simulink model "simulink_controll_attitude_5kg"  (R2015a)
settings: Solver=ode45  StartTime=0.0  StopTime=40  RelTol=1e-3
libraries: fuzblock x4
settings Model: Creator=Marcos  LastModifiedBy=Marcos

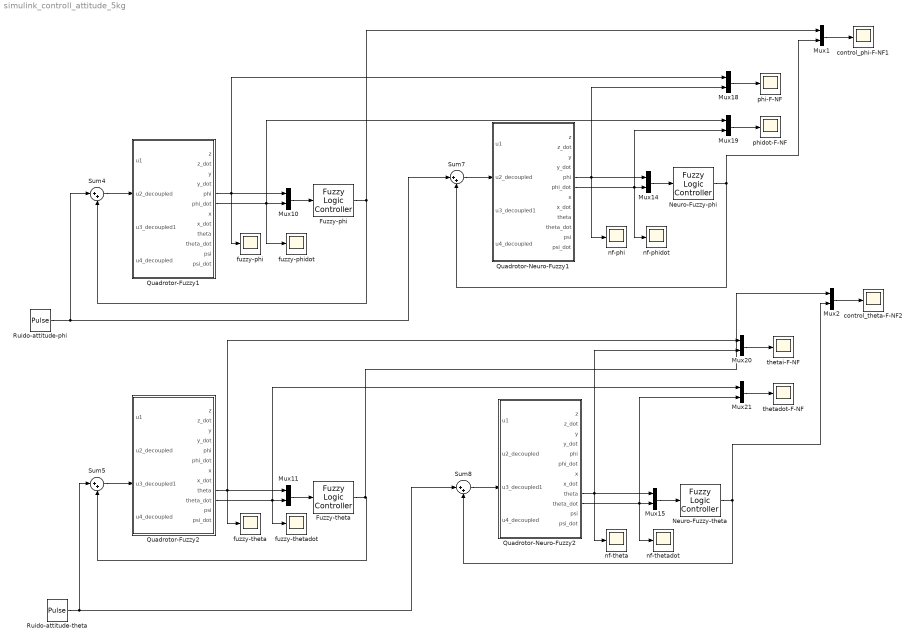
== system simulink_controll_attitude_5kg ==
  Fuzzy-phi : fuzblock/Fuzzy Logic  Controller  fis='fis_attitude.fis'
  Fuzzy-theta : fuzblock/Fuzzy Logic  Controller  fis='fis_attitude.fis'
  Mux{1..2,10..11,14..15,18..21} (10 alike) : Mux  Inputs=2
  Neuro-Fuzzy-phi : fuzblock/Fuzzy Logic  Controller  fis='anfis_attitude.fis'
  Neuro-Fuzzy-theta : fuzblock/Fuzzy Logic  Controller  fis='anfis_attitude.fis'
  Quadrotor-Fuzzy1 : Subsystem
  Quadrotor-Fuzzy2 : Subsystem
  Quadrotor-Neuro-Fuzzy1 : Subsystem
  Quadrotor-Neuro-Fuzzy2 : Subsystem
  Ruido-attitude-phi : DiscretePulseGenerator  PulseType=Time based  Amplitude=20  Period=40  PulseWidth=0.05
  Ruido-attitude-theta : DiscretePulseGenerator  PulseType=Time based  Amplitude=20  Period=40  PulseWidth=0.05
  Sum{4..5,7..8} (4 alike) : Sum  Inputs=|++
  control_phi-F-NF1 : Scope
      settings: SaveName=control_phi5
  control_theta-F-NF2 : Scope
      settings: SaveName=control_theta5
  fuzzy-phi : Scope
      settings: SaveName=ScopeData19
  fuzzy-phidot : Scope
      settings: SaveName=ScopeData20
  fuzzy-theta : Scope
      settings: SaveName=ScopeData21
  fuzzy-thetadot : Scope
      settings: SaveName=ScopeData22
  nf-phi : Scope
      settings: SaveName=ScopeData25
  nf-phidot : Scope
      settings: SaveName=ScopeData26
  nf-theta : Scope
      settings: SaveName=ScopeData27
  nf-thetadot : Scope
      settings: SaveName=ScopeData28
  phi-F-NF : Scope
      settings: SaveName=phi5
  phidot-F-NF : Scope
      settings: SaveName=phidot5
  thetadot-F-NF : Scope
      settings: SaveName=thetadot5
  thetai-F-NF : Scope
      settings: SaveName=theta5
  wires:
  Mux10/1 -> Fuzzy-phi/1
  Quadrotor-Fuzzy1/5(phi) -> Mux18/1, fuzzy-phi/1, Mux10/1
  Sum4/1 -> Quadrotor-Fuzzy1/2(u2_decoupled)
  Fuzzy-phi/1 -> Sum4/2, Mux1/1
  Quadrotor-Fuzzy1/6(phi_dot) -> Mux19/1, fuzzy-phidot/1, Mux10/2
  Quadrotor-Fuzzy2/9(theta) -> Mux20/1, fuzzy-theta/1, Mux11/1
  Sum5/1 -> Quadrotor-Fuzzy2/3(u3_decoupled1)
  Fuzzy-theta/1 -> Mux2/1, Sum5/2
  Quadrotor-Fuzzy2/10(theta_dot) -> fuzzy-thetadot/1, Mux21/1, Mux11/2
  Mux11/1 -> Fuzzy-theta/1
  Mux14/1 -> Neuro-Fuzzy-phi/1
  Ruido-attitude-phi/1 -> Sum7/1, Sum4/1
  Quadrotor-Neuro-Fuzzy1/5(phi) -> Mux18/2, nf-phi/1, Mux14/1
  Sum7/1 -> Quadrotor-Neuro-Fuzzy1/2(u2_decoupled)
  Neuro-Fuzzy-phi/1 -> Mux1/2, Sum7/2
  Quadrotor-Neuro-Fuzzy1/6(phi_dot) -> Mux19/2, nf-phidot/1, Mux14/2
  Ruido-attitude-theta/1 -> Sum8/1, Sum5/1
  Quadrotor-Neuro-Fuzzy2/9(theta) -> Mux20/2, nf-theta/1, Mux15/1
  Sum8/1 -> Quadrotor-Neuro-Fuzzy2/3(u3_decoupled1)
  Neuro-Fuzzy-theta/1 -> Mux2/2, Sum8/2
  Quadrotor-Neuro-Fuzzy2/10(theta_dot) -> Mux21/2, nf-thetadot/1, Mux15/2
  Mux15/1 -> Neuro-Fuzzy-theta/1
  Mux20/1 -> thetai-F-NF/1
  Mux21/1 -> thetadot-F-NF/1
  Mux18/1 -> phi-F-NF/1
  Mux19/1 -> phidot-F-NF/1
  Mux1/1 -> control_phi-F-NF1/1
  Mux2/1 -> control_theta-F-NF2/1

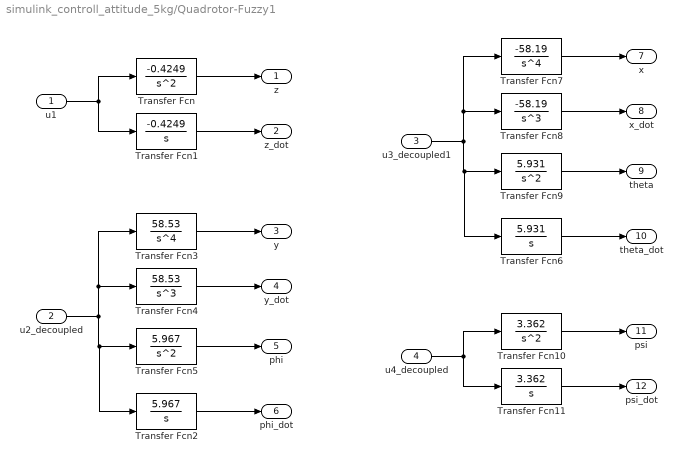
== system simulink_controll_attitude_5kg/Quadrotor-Fuzzy1 ==
  u1 : Inport
  u2_decoupled : Inport  Port=2
  u3_decoupled1 : Inport  Port=3
  u4_decoupled : Inport  Port=4
  Transfer Fcn : TransferFcn  Numerator=[-0.4249]  Denominator=[1 0 0]
  Transfer Fcn1 : TransferFcn  Numerator=[-0.4249]  Denominator=[1 0]
  Transfer Fcn10 : TransferFcn  Numerator=[3.362]  Denominator=[1 0 0]
  Transfer Fcn11 : TransferFcn  Numerator=[3.362]  Denominator=[1 0]
  Transfer Fcn2 : TransferFcn  Numerator=[5.967]  Denominator=[1 0]
  Transfer Fcn3 : TransferFcn  Numerator=[58.53]  Denominator=[1 0 0 0 0]
  Transfer Fcn4 : TransferFcn  Numerator=[58.53]  Denominator=[1 0 0 0]
  Transfer Fcn5 : TransferFcn  Numerator=[5.967]  Denominator=[1 0 0]
  Transfer Fcn6 : TransferFcn  Numerator=[5.931]  Denominator=[1 0]
  Transfer Fcn7 : TransferFcn  Numerator=[-58.19]  Denominator=[1 0 0 0 0]
  Transfer Fcn8 : TransferFcn  Numerator=[-58.19]  Denominator=[1 0 0 0]
  Transfer Fcn9 : TransferFcn  Numerator=[5.931]  Denominator=[1 0 0]
  z : Outport
  z_dot : Outport  Port=2
  y : Outport  Port=3
  y_dot : Outport  Port=4
  phi : Outport  Port=5
  phi_dot : Outport  Port=6
  x : Outport  Port=7
  x_dot : Outport  Port=8
  theta : Outport  Port=9
  theta_dot : Outport  Port=10
  psi : Outport  Port=11
  psi_dot : Outport  Port=12
  wires:
  Transfer Fcn/1 -> z/1
  u1/1 -> Transfer Fcn/1, Transfer Fcn1/1
  Transfer Fcn1/1 -> z_dot/1
  Transfer Fcn3/1 -> y/1
  u2_decoupled/1 -> Transfer Fcn3/1, Transfer Fcn4/1, Transfer Fcn2/1, Transfer Fcn5/1
  Transfer Fcn4/1 -> y_dot/1
  Transfer Fcn5/1 -> phi/1
  Transfer Fcn2/1 -> phi_dot/1
  Transfer Fcn7/1 -> x/1
  u3_decoupled1/1 -> Transfer Fcn7/1, Transfer Fcn8/1, Transfer Fcn6/1, Transfer Fcn9/1
  Transfer Fcn8/1 -> x_dot/1
  Transfer Fcn9/1 -> theta/1
  Transfer Fcn6/1 -> theta_dot/1
  Transfer Fcn10/1 -> psi/1
  u4_decoupled/1 -> Transfer Fcn10/1, Transfer Fcn11/1
  Transfer Fcn11/1 -> psi_dot/1

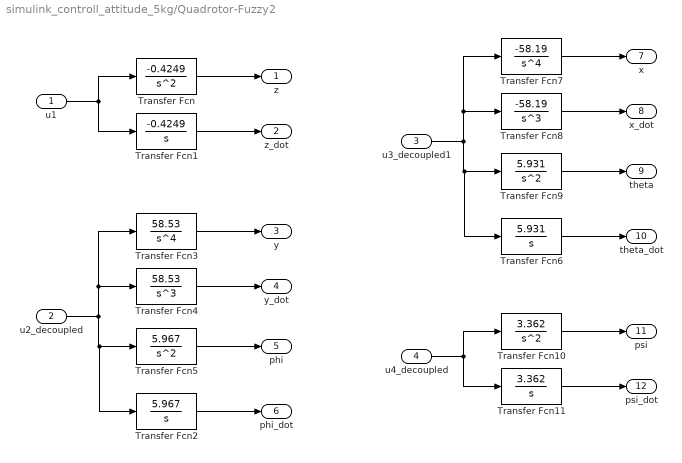
== system simulink_controll_attitude_5kg/Quadrotor-Fuzzy2 ==
  u1 : Inport
  u2_decoupled : Inport  Port=2
  u3_decoupled1 : Inport  Port=3
  u4_decoupled : Inport  Port=4
  Transfer Fcn : TransferFcn  Numerator=[-0.4249]  Denominator=[1 0 0]
  Transfer Fcn1 : TransferFcn  Numerator=[-0.4249]  Denominator=[1 0]
  Transfer Fcn10 : TransferFcn  Numerator=[3.362]  Denominator=[1 0 0]
  Transfer Fcn11 : TransferFcn  Numerator=[3.362]  Denominator=[1 0]
  Transfer Fcn2 : TransferFcn  Numerator=[5.967]  Denominator=[1 0]
  Transfer Fcn3 : TransferFcn  Numerator=[58.53]  Denominator=[1 0 0 0 0]
  Transfer Fcn4 : TransferFcn  Numerator=[58.53]  Denominator=[1 0 0 0]
  Transfer Fcn5 : TransferFcn  Numerator=[5.967]  Denominator=[1 0 0]
  Transfer Fcn6 : TransferFcn  Numerator=[5.931]  Denominator=[1 0]
  Transfer Fcn7 : TransferFcn  Numerator=[-58.19]  Denominator=[1 0 0 0 0]
  Transfer Fcn8 : TransferFcn  Numerator=[-58.19]  Denominator=[1 0 0 0]
  Transfer Fcn9 : TransferFcn  Numerator=[5.931]  Denominator=[1 0 0]
  z : Outport
  z_dot : Outport  Port=2
  y : Outport  Port=3
  y_dot : Outport  Port=4
  phi : Outport  Port=5
  phi_dot : Outport  Port=6
  x : Outport  Port=7
  x_dot : Outport  Port=8
  theta : Outport  Port=9
  theta_dot : Outport  Port=10
  psi : Outport  Port=11
  psi_dot : Outport  Port=12
  wires:
  Transfer Fcn/1 -> z/1
  u1/1 -> Transfer Fcn/1, Transfer Fcn1/1
  Transfer Fcn1/1 -> z_dot/1
  Transfer Fcn3/1 -> y/1
  u2_decoupled/1 -> Transfer Fcn3/1, Transfer Fcn4/1, Transfer Fcn2/1, Transfer Fcn5/1
  Transfer Fcn4/1 -> y_dot/1
  Transfer Fcn5/1 -> phi/1
  Transfer Fcn2/1 -> phi_dot/1
  Transfer Fcn7/1 -> x/1
  u3_decoupled1/1 -> Transfer Fcn7/1, Transfer Fcn8/1, Transfer Fcn6/1, Transfer Fcn9/1
  Transfer Fcn8/1 -> x_dot/1
  Transfer Fcn9/1 -> theta/1
  Transfer Fcn6/1 -> theta_dot/1
  Transfer Fcn10/1 -> psi/1
  u4_decoupled/1 -> Transfer Fcn10/1, Transfer Fcn11/1
  Transfer Fcn11/1 -> psi_dot/1

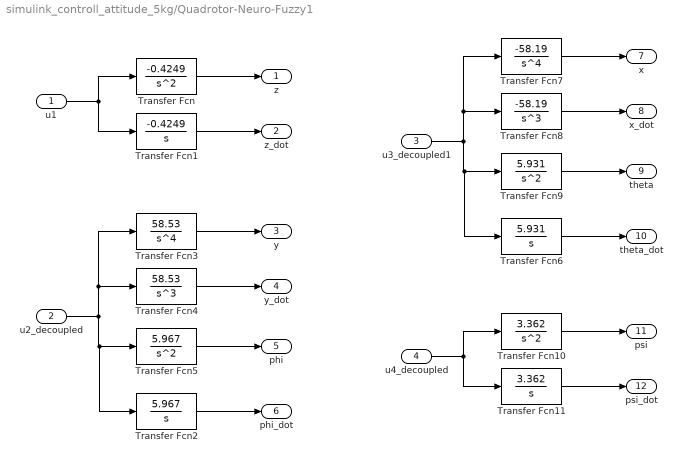
== system simulink_controll_attitude_5kg/Quadrotor-Neuro-Fuzzy1 ==
  u1 : Inport
  u2_decoupled : Inport  Port=2
  u3_decoupled1 : Inport  Port=3
  u4_decoupled : Inport  Port=4
  Transfer Fcn : TransferFcn  Numerator=[-0.4249]  Denominator=[1 0 0]
  Transfer Fcn1 : TransferFcn  Numerator=[-0.4249]  Denominator=[1 0]
  Transfer Fcn10 : TransferFcn  Numerator=[3.362]  Denominator=[1 0 0]
  Transfer Fcn11 : TransferFcn  Numerator=[3.362]  Denominator=[1 0]
  Transfer Fcn2 : TransferFcn  Numerator=[5.967]  Denominator=[1 0]
  Transfer Fcn3 : TransferFcn  Numerator=[58.53]  Denominator=[1 0 0 0 0]
  Transfer Fcn4 : TransferFcn  Numerator=[58.53]  Denominator=[1 0 0 0]
  Transfer Fcn5 : TransferFcn  Numerator=[5.967]  Denominator=[1 0 0]
  Transfer Fcn6 : TransferFcn  Numerator=[5.931]  Denominator=[1 0]
  Transfer Fcn7 : TransferFcn  Numerator=[-58.19]  Denominator=[1 0 0 0 0]
  Transfer Fcn8 : TransferFcn  Numerator=[-58.19]  Denominator=[1 0 0 0]
  Transfer Fcn9 : TransferFcn  Numerator=[5.931]  Denominator=[1 0 0]
  z : Outport
  z_dot : Outport  Port=2
  y : Outport  Port=3
  y_dot : Outport  Port=4
  phi : Outport  Port=5
  phi_dot : Outport  Port=6
  x : Outport  Port=7
  x_dot : Outport  Port=8
  theta : Outport  Port=9
  theta_dot : Outport  Port=10
  psi : Outport  Port=11
  psi_dot : Outport  Port=12
  wires:
  Transfer Fcn/1 -> z/1
  u1/1 -> Transfer Fcn/1, Transfer Fcn1/1
  Transfer Fcn1/1 -> z_dot/1
  Transfer Fcn3/1 -> y/1
  u2_decoupled/1 -> Transfer Fcn3/1, Transfer Fcn4/1, Transfer Fcn2/1, Transfer Fcn5/1
  Transfer Fcn4/1 -> y_dot/1
  Transfer Fcn5/1 -> phi/1
  Transfer Fcn2/1 -> phi_dot/1
  Transfer Fcn7/1 -> x/1
  u3_decoupled1/1 -> Transfer Fcn7/1, Transfer Fcn8/1, Transfer Fcn6/1, Transfer Fcn9/1
  Transfer Fcn8/1 -> x_dot/1
  Transfer Fcn9/1 -> theta/1
  Transfer Fcn6/1 -> theta_dot/1
  Transfer Fcn10/1 -> psi/1
  u4_decoupled/1 -> Transfer Fcn10/1, Transfer Fcn11/1
  Transfer Fcn11/1 -> psi_dot/1

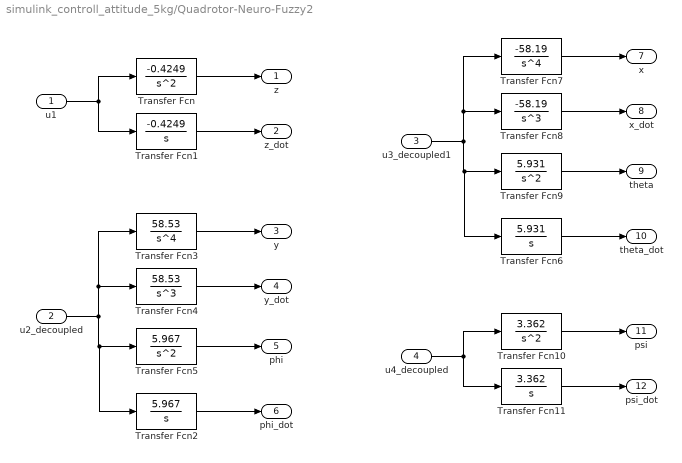
== system simulink_controll_attitude_5kg/Quadrotor-Neuro-Fuzzy2 ==
  u1 : Inport
  u2_decoupled : Inport  Port=2
  u3_decoupled1 : Inport  Port=3
  u4_decoupled : Inport  Port=4
  Transfer Fcn : TransferFcn  Numerator=[-0.4249]  Denominator=[1 0 0]
  Transfer Fcn1 : TransferFcn  Numerator=[-0.4249]  Denominator=[1 0]
  Transfer Fcn10 : TransferFcn  Numerator=[3.362]  Denominator=[1 0 0]
  Transfer Fcn11 : TransferFcn  Numerator=[3.362]  Denominator=[1 0]
  Transfer Fcn2 : TransferFcn  Numerator=[5.967]  Denominator=[1 0]
  Transfer Fcn3 : TransferFcn  Numerator=[58.53]  Denominator=[1 0 0 0 0]
  Transfer Fcn4 : TransferFcn  Numerator=[58.53]  Denominator=[1 0 0 0]
  Transfer Fcn5 : TransferFcn  Numerator=[5.967]  Denominator=[1 0 0]
  Transfer Fcn6 : TransferFcn  Numerator=[5.931]  Denominator=[1 0]
  Transfer Fcn7 : TransferFcn  Numerator=[-58.19]  Denominator=[1 0 0 0 0]
  Transfer Fcn8 : TransferFcn  Numerator=[-58.19]  Denominator=[1 0 0 0]
  Transfer Fcn9 : TransferFcn  Numerator=[5.931]  Denominator=[1 0 0]
  z : Outport
  z_dot : Outport  Port=2
  y : Outport  Port=3
  y_dot : Outport  Port=4
  phi : Outport  Port=5
  phi_dot : Outport  Port=6
  x : Outport  Port=7
  x_dot : Outport  Port=8
  theta : Outport  Port=9
  theta_dot : Outport  Port=10
  psi : Outport  Port=11
  psi_dot : Outport  Port=12
  wires:
  Transfer Fcn/1 -> z/1
  u1/1 -> Transfer Fcn/1, Transfer Fcn1/1
  Transfer Fcn1/1 -> z_dot/1
  Transfer Fcn3/1 -> y/1
  u2_decoupled/1 -> Transfer Fcn3/1, Transfer Fcn4/1, Transfer Fcn2/1, Transfer Fcn5/1
  Transfer Fcn4/1 -> y_dot/1
  Transfer Fcn5/1 -> phi/1
  Transfer Fcn2/1 -> phi_dot/1
  Transfer Fcn7/1 -> x/1
  u3_decoupled1/1 -> Transfer Fcn7/1, Transfer Fcn8/1, Transfer Fcn6/1, Transfer Fcn9/1
  Transfer Fcn8/1 -> x_dot/1
  Transfer Fcn9/1 -> theta/1
  Transfer Fcn6/1 -> theta_dot/1
  Transfer Fcn10/1 -> psi/1
  u4_decoupled/1 -> Transfer Fcn10/1, Transfer Fcn11/1
  Transfer Fcn11/1 -> psi_dot/1
